simulink library "tqd"  (R2021b)
settings: Solver=VariableStepAuto  StartTime=0.0  StopTime=10.0  RelTol=1e-3
undefined symbols (not defined in the file or in its folder): ATQD_APSDecReq_X_kph, ATQD_APSDecReq_Y_mps2, ATQD_APSDecReqCMD_X_kph, ATQD_APSDecReqTs_X_pct, ATQD_APSDecTimeGain_X_Deg, ATQD_APSDecTimeGain_Y_s, ATQD_APSReqLowSpd_X_Deg, ATQD_AutoHoldReleaseBPS_X_Deg, ATQD_AWDLoadTrqnsGain_X_kg, ATQD_AWDLoadTrqnsGain_Y_pct, ATQD_BOSEnBPSPosn_X_kph, ATQD_BOSMap_X_rpm, ATQD_BOSMap_Y_pct, ATQD_CreepBaseTqD_X_kph, ATQD_CreepBaseTqD_Y_Deg, ATQD_CreepBaseTqR_X_kph, ATQD_CreepBaseTqR_Y_Deg, ATQD_CreepBPSDisPosn_X_Deg, ATQD_CreepBPSDisPosnR_X_Deg, ATQD_CreepBPSEnPosn_X_Deg, ATQD_CreepBPSEnPosnR_X_Deg, ATQD_CreepDeltaTq_X_kph, ATQD_CreepIterm_X_kph, ATQD_CreepIterm_Y_kph, ATQD_CreepItermMaxLimit_X_pct, ATQD_CreepPreloadTime_X_kph, ATQD_CreepPreloadTq_X_kph, ATQD_CreepPreloadTq_Y_s, ATQD_CreepProtTq_X_Deg, ATQD_CreepPterm_X_kph, ATQD_CreepPterm_Y_kph, ATQD_ECOTqMapD_X_rpm, ATQD_ECOTqMapD_Y_pct, ATQD_EOPDTqMapDCon_X_rpm, ATQD_EOPDTqMapDCon_Y_Deg, ATQD_EstInitVehWeight_X_c, ATQD_LHMRollGenMapD_X_rpm, ATQD_LHMRollGenMapD_Y_rpm, ATQD_LHMTqMapD_X_rpm, ATQD_LHMTqMapD_Y_pct, ATQD_NL1TqMapD_X_rpm, ATQD_NL1TqMapD_Y_pct, ATQD_NOPDTqMapDCon_X_rpm, ATQD_NOPDTqMapDCon_Y_Deg, ATQD_NRMRrEDUSpRat_X_rpm, ATQD_NRMRrEDUSpRat_Y_Nm, ATQD_OPDHoldDownRelDelay_X_Deg, ATQD_OPDHoldEnSpd_X_Deg, ATQD_OPDHoldRelDetTime_X_Deg, ATQD_OPDHoldReleaseTq_X_Deg, ATQD_OrigPedTqLowLim_X_Deg, ATQD_OrigPedTqLowLim_Y_pct, ATQD_PedalMapClimbUpLim_X_rpm, ATQD_PedalMapClimbUpLim_Y_Deg, ATQD_PreLoadTq_X_s, ATQD_RollGenMapEL1_X_rpm, ATQD_RollGenMapEL1_Y_rpm, ATQD_SL1TqMapD_X_rpm, ATQD_SL1TqMapD_Y_pct, ATQD_SlideRegenTqGain_X_Gps ... (+487)
libraries: hcu_lib x83, simulink x73, tqr x1
(part 9 of 19)

== system tqd/TQD/TorqueDemand/Signal_convert/SWC2_Subsystem/L_ScrollPress Behavior ==
  note: If press time more then Long press's limit then go Long press only. Else go short press only. Else if no press.
  note: Long press or Short press
  VTQD_SWC2LScrollPressSta_flg : Inport
  TASK_TIME : Inport  Port=2
  AND : Logic  AllPortsSameDT=off  OutDataTypeStr=boolean
  Constant10 : Constant  Value=FALSE
  Constant3 : Constant  Value=KTQD_SpdModeShortPLim_s
  Constant7 : Constant  Value=FALSE
  Default 3 sec : Constant  Value=KTQD_SpdModeLongPLim_s
  DelayEnable_LONG_PRESS : hcu_lib/Basic_Blocks/DelayEnable
  DelayEnable_SHORT_PRESS : hcu_lib/Basic_Blocks/DelayEnable
  Detect Decrease1 : simulink/Logic and Bit Operations/Detect Decrease  vinit=0.0  OutDataTypeStr=boolean
  Detect Decrease2 : simulink/Logic and Bit Operations/Detect Decrease  vinit=0.0  OutDataTypeStr=boolean
  Detect Increase : simulink/Logic and Bit Operations/Detect Increase  vinit=0.0  OutDataTypeStr=boolean
  Switch1 : Switch  Criteria=u2 > Threshold
  Switch2 : Switch  Criteria=u2 ~= 0
  VTQD_LScrollPressShort_flg : Outport
  "VTQD_LScrollPressLong_flg\t" : Outport  Port=2
  wires:
  Detect Increase/1 -> "VTQD_LScrollPressLong_flg\t"/1
  [TASK_TIME] -> DelayEnable_LONG_PRESS/3
  Default 3 sec/1 -> DelayEnable_LONG_PRESS/2
  [TASK_TIME] -> DelayEnable_SHORT_PRESS/3
  Constant3/1 -> DelayEnable_SHORT_PRESS/2
  DelayEnable_SHORT_PRESS/1 -> Detect Decrease2/1
  Constant7/1 -> Switch1/3
  DelayEnable_LONG_PRESS/1 -> Switch1/1, Switch1/2
  [Short_press_falling_Edge] -> AND/1
  [Long_press] -> Detect Decrease1/1, Detect Increase/1
  Constant10/1 -> Switch2/1
  [Short_press_falling_Edge] -> Switch2/3
  [VTQD_SWC2LScrollPressSta_flg] -> DelayEnable_SHORT_PRESS/1, DelayEnable_LONG_PRESS/1
  AND/1 -> Switch2/2
  Switch2/1 -> VTQD_LScrollPressShort_flg/1
  VTQD_SWC2LScrollPressSta_flg/1 -> [VTQD_SWC2LScrollPressSta_flg]
  Detect Decrease1/1 -> AND/2
  Detect Decrease2/1 -> [Short_press_falling_Edge]
  Switch1/1 -> [Long_press]
  TASK_TIME/1 -> [TASK_TIME]

== system tqd/TQD/TorqueDemand/Signal_convert/SWC2_Subsystem/Road Speed Limit Convert ==
  VINP_ADASSLIFSpdLim_enum : Inport
  VINP_IVIISAOffsetSpd_enum : Inport  Port=2
  VTQD_IVIISAOffsetSpdCHOOSE_flg : Inport  Port=3
  VINP_Distanceunit_flg : Inport  Port=4
  VTQD_ShiftGearPosn_enum : Inport  Port=5
  " 20" : Constant  Value=KTQD_ACCActiveMetSpdLoMPH_mph
  " 30kph" : Constant  Value=KTQD_ACCActiveMetSpdLo_kph
  AND{,1..3} (4 alike) : Logic  AllPortsSameDT=off  OutDataTypeStr=boolean
  Add{,1..3} (4 alike) : Sum  Inputs=+-
  Add4 : Sum
  Constant{,17..18,20} (4 alike) : Constant  Value=0x11  OutDataTypeStr=uint8
  Constant1 : Constant  Value=10  OutDataTypeStr=single
  Constant10 : Constant  Value=15  OutDataTypeStr=single
  Constant{11,13..15} (4 alike) : Constant  Value=ZERO_FLOAT  OutDataTypeStr=single
  Constant12 : Constant  Value=ENUM_GEARPOSNTOCAN_D  OutDataTypeStr=uint8
  Constant16 : Constant  Value=KTQD_SpdLimOffsetOn_flg  OutDataTypeStr=single
  Constant19 : Constant  Value=MPH2KPH  OutDataTypeStr=uint8
  Constant2 : Constant  Value=0x10  OutDataTypeStr=uint8
  Constant21 : Constant  Value=KPH2MPH  OutDataTypeStr=uint8
  Constant{3,7..9} (4 alike) : Constant  Value=5  OutDataTypeStr=single
  Constant4 : Constant  Value=0x0  OutDataTypeStr=uint8
  Constant5 : Constant  Value=0x9  OutDataTypeStr=uint8
  Constant6 : Constant  Value=0x9  OutDataTypeStr=uint8
  Data Type Conversion{,1..3} (4 alike) : DataTypeConversion  OutDataTypeStr=single
  Delay : Delay  DelayLength=1
  Divide : Product  Inputs=**
  Divide1 : Product  Inputs=**
  Equal : RelationalOperator  Operator=~=  OutDataTypeStr=boolean  RndMeth=Simplest
  Equal1 : RelationalOperator  Operator===  OutDataTypeStr=boolean  RndMeth=Simplest
  Max : MinMax  Function=max  Inputs=2
  NOT : Logic  Operator=NOT  AllPortsSameDT=off  OutDataTypeStr=boolean
  NOT1 : Logic  Operator=NOT  AllPortsSameDT=off  OutDataTypeStr=boolean
  Product{,1..3} (4 alike) : Product
  Relational Operator{,1,3..5} (5 alike) : RelationalOperator  OutDataTypeStr=boolean  RndMeth=Simplest
  Relational Operator2 : RelationalOperator  Operator=>  OutDataTypeStr=boolean  RndMeth=Simplest
  Switch{,1..9} (10 alike) : Switch  Criteria=u2 > Threshold
  VTQD_RoadSpdLim_raw32 : Outport
  wires:
  VINP_ADASSLIFSpdLim_enum/1 -> [VINP_ADASSLIFSpdLim_enum]
  VINP_IVIISAOffsetSpd_enum/1 -> [VINP_IVIISAOffsetSpd_enum]
  [VINP_ADASSLIFSpdLim_enum] -> Relational Operator/1
  Relational Operator/1 -> Switch/2
  Constant/1 -> Relational Operator/2
  [VINP_ADASSLIFSpdLim_enum] -> Data Type Conversion/1
  Data Type Conversion/1 -> Product/1
  Constant1/1 -> Product/2
  Product/1 -> Switch/3
  [VINP_ADASSLIFSpdLim_enum] -> Add/1
  Constant2/1 -> Add/2
  Product1/1 -> Switch/1
  Constant3/1 -> Product1/2
  Add/1 -> Data Type Conversion1/1
  Data Type Conversion1/1 -> Product1/1
  Equal/1 -> Switch1/2
  Constant4/1 -> Equal/2
  Switch/1 -> Switch1/1
  Switch5/1 -> [VTQD_CalRoadSpdLim_raw32], Delay/1  "VTQD_CalRoadSpdLim_raw32"
  [VINP_IVIISAOffsetSpd_enum] -> Relational Operator1/1
  Constant5/1 -> Relational Operator1/2
  Relational Operator1/1 -> Switch2/2
  Data Type Conversion2/1 -> Product2/1
  [VINP_IVIISAOffsetSpd_enum] -> Add1/1
  Constant6/1 -> Add1/2
  Add1/1 -> Data Type Conversion2/1
  Constant7/1 -> Product2/2
  Product2/1 -> Add2/1
  Constant8/1 -> Add2/2
  [VINP_IVIISAOffsetSpd_enum] -> Data Type Conversion3/1
  Constant9/1 -> Product3/2
  Data Type Conversion3/1 -> Product3/1
  Constant10/1 -> Add3/2
  Product3/1 -> Add3/1
  Add3/1 -> Switch2/3
  Add2/1 -> Switch2/1
  VTQD_IVIISAOffsetSpdCHOOSE_flg/1 -> [VTQD_IVIISAOffsetSpdCHOOSE_flg]
  Switch2/1 -> Switch3/1
  Constant11/1 -> Switch3/3
  Switch3/1 -> [VTQD_CalRoadSpdLimOffSet_c]  "VTQD_CalRoadSpdLimOffSet_c"
  Switch6/1 -> Add4/2
  [VTQD_CalRoadSpdLim_raw32] -> Add4/1
  [VTQD_RoadSpdLim_raw32] -> VTQD_RoadSpdLim_raw32/1
  [VTQD_IVIISAOffsetSpdCHOOSE_flg] -> AND/1
  " 20"/1 -> Switch4/1
  " 30kph"/1 -> Switch4/3
  [VINP_Distanceunit_flg] -> Switch4/2
  VINP_Distanceunit_flg/1 -> [VINP_Distanceunit_flg]
  Delay/1 -> Switch1/3
  Switch4/1 -> Max/1
  Max/1 -> [VTQD_RoadSpdLim_raw32]  "VTQD_RoadSpdLim_raw32"
  Add4/1 -> [VTQD_SpdLimAftOffset_raw32]  "VTQD_SpdLimAftOffset_raw32"
  [VINP_ADASSLIFSpdLim_enum] -> Equal/1
  Equal1/1 -> Switch5/2
  Constant12/1 -> Equal1/2
  Switch1/1 -> Switch5/1
  Constant13/1 -> Switch5/3
  VTQD_ShiftGearPosn_enum/1 -> [VTQD_ShiftGearPosn_enum]
  [VTQD_ShiftGearPosn_enum] -> Equal1/1
  [VTQD_CalRoadSpdLimOffSet_c] -> Relational Operator2/1, Switch6/1
  Relational Operator2/1 -> Switch6/2
  Constant14/1 -> Relational Operator2/2
  Constant15/1 -> Switch6/3
  AND/1 -> Switch3/2
  Constant16/1 -> AND/2
  Constant17/1 -> Relational Operator3/2
  [VINP_ADASSLIFSpdLim_enum] -> Relational Operator3/1
  Relational Operator3/1 -> AND1/2
  [VINP_Distanceunit_flg] -> AND1/1
  AND1/1 -> Switch7/2
  Switch7/1 -> Max/2
  [VTQD_SpdLimAftOffset_raw32] -> Switch7/1
  AND2/1 -> Switch8/2
  [VINP_Distanceunit_flg] -> NOT/1
  Relational Operator4/1 -> AND2/2
  [VINP_ADASSLIFSpdLim_enum] -> Relational Operator4/1
  Constant18/1 -> Relational Operator4/2
  Switch8/1 -> Switch7/3
  NOT/1 -> AND2/1
  [VTQD_SpdLimAftOffset_raw32] -> Divide/1
  Divide/1 -> Switch8/1
  Constant19/1 -> Divide/2
  AND3/1 -> Switch9/2
  [VINP_Distanceunit_flg] -> AND3/1
  Relational Operator5/1 -> NOT1/1
  [VINP_ADASSLIFSpdLim_enum] -> Relational Operator5/1
  Constant20/1 -> Relational Operator5/2
  Switch9/1 -> Switch8/3
  NOT1/1 -> AND3/2
  Constant21/1 -> Divide1/2
  [VTQD_SpdLimAftOffset_raw32] -> Divide1/1
  Divide1/1 -> Switch9/1
  [VTQD_SpdLimAftOffset_raw32] -> Switch9/3

== system tqd/TQD/TorqueDemand/Signal_convert/SWC2_Subsystem/Speed Setting Mode ==
  note: Botton logic
  note: INPUT Signal
  note: PWRSTA and DRIVE GEAR GOOD
  note: OUTPUT SET SPEED
  VPMM_PowerSta_enum : Inport
  VTQD_ShiftGearPosn_enum : Inport  Port=2
  VTQD_SpdCtrlMode_enum : Inport  Port=3
  VINP_ADASACCSta_enum : Inport  Port=4
  VVMC_CCCtrlSta_enum : Inport  Port=5
  VVMC_MSACtrlSta_enum : Inport  Port=6
  VINP_ADASSLIFSpdLim_enum : Inport  Port=7
  VTQD_SWC2ScrollUpSta_flg : Inport  Port=8
  VTQD_SWC2ScrollDownSta_flg : Inport  Port=9
  task_time_s : Inport  Port=10
  VVMC_LVDAACCStatusInformation_flg : Inport  Port=11
  VVMC_ACCObjDist_m : Inport  Port=12
  VTQD_SpdLim4SetSpd_raw32 : Inport  Port=13
  VINP_Distanceunit_flg : Inport  Port=14
  VTQD_SWC2ResUpSta_flg : Inport  Port=15
  VTQD_SWC2SetDownSta_flg : Inport  Port=16
  VINP_SmartEcoModeSW_flg : Inport  Port=17
  VVMC_SetACCDisableAPS_flg : Inport  Port=18
  VINP_IVIACCAdaptiveSta_flg : Inport  Port=19
  VTQD_Set2MeterSpd_flg : Inport  Port=20
  VTQD_SetRoadSpdLim_flg : Inport  Port=21
  VTQD_LScrollPressShort_flg : Inport  Port=22
  VVMC_MeterIndSpeed_raw32 : Inport  Port=23
  ACC Speed Setting ON : Subsystem  TreatAsAtomicUnit=on
  AND{,1..3,5,8} (6 alike) : Logic  AllPortsSameDT=off  OutDataTypeStr=boolean
  AND6 : Logic  Inputs=3  AllPortsSameDT=off  OutDataTypeStr=boolean
  AND7 : Logic  Operator=OR  AllPortsSameDT=off  OutDataTypeStr=boolean
  CC Speed Setting ON : Subsystem  TreatAsAtomicUnit=on
  Constant : Constant  Value=ZERO_INT
  Constant1 : Constant  Value=ENUM_SPDCTRLMODE_CC
  Constant10 : Constant  Value=ENUM_SPDCTRLMODE_ISA
  Constant11 : Constant  Value=ENUM_SPDCTRLMODE_OFF
  Constant12 : Constant  Value=KTQD_SetSpdDeltaLongFit_kph
  Constant13 : Constant  Value=ZERO_INT
  Constant14 : Constant  Value=KTQD_SmartEcoLimitSpd_kph
  Constant15 : Constant  Value=KTQD_SmartEcoLimitSpd_mph
  Constant16 : Constant  Value=KTQD_SmartEcoLimitSpd_kph
  Constant17 : Constant  Value=KTQD_SmartEcoLimitSpd_mph
  Constant18 : Constant  Value=KTQD_SmartEcoLimitSpd_kph
  Constant19 : Constant  Value=KTQD_SmartEcoLimitSpd_mph
  Constant2 : Constant  Value=ENUM_POWERSTA_READY
  Constant3 : Constant  Value=ENUM_SPDCTRLMODE_ACC
  Constant4 : Constant  Value=ENUM_GEARPOSNTOCAN_D
  Constant5 : Constant  Value=ENUM_SPDCTRLMODE_MSA
  Constant6 : Constant  Value=ENUM_SPDCTRLMODE_ISA
  Constant7 : Constant  Value=ENUM_SPDCTRLMODE_ACC
  Constant8 : Constant  Value=ENUM_SPDCTRLMODE_CC
  Constant9 : Constant  Value=ENUM_SPDCTRLMODE_MSA
  Data Type Conversion : DataTypeConversion  OutDataTypeStr=uint8
  Delay : Delay  DelayLength=1
  Else Speed Setting On : Subsystem  TreatAsAtomicUnit=on
  Equal{1..11} (11 alike) : RelationalOperator  Operator===  OutDataTypeStr=boolean  RndMeth=Simplest
  ISA Speed Setting ON : Subsystem  TreatAsAtomicUnit=on
  If : If  NumInputs=4  IfExpression=u1 ~= 0  ElseIfExpressions=u2 ~= 0, u3~= 0, u4~= 0
  MSA Speed Setting ON : Subsystem  TreatAsAtomicUnit=on
  OR : Logic  Operator=OR  AllPortsSameDT=off  OutDataTypeStr=boolean
  Relational Operator : RelationalOperator  OutDataTypeStr=boolean  RndMeth=Simplest
  Relational Operator1 : RelationalOperator  OutDataTypeStr=boolean  RndMeth=Simplest
  Relational Operator2 : RelationalOperator  OutDataTypeStr=boolean  RndMeth=Simplest
  Rem : Math  Operator=rem  SaturateOnIntegerOverflow=on
  SWC2ScrollDownSta : Subsystem
  SWC2ScrollUpSta : Subsystem
  Switch{,1..4} (5 alike) : Switch  Criteria=u2 ~= 0
  Switch5 : Switch  Criteria=u2 > Threshold
  Switch6 : Switch  Criteria=u2 > Threshold
  Switch7 : Switch  Criteria=u2 > Threshold
  VTQD_SetSpd_kph : Outport
  VTQD_SWC2ScrollUpSta_enum : Outport  Port=2
  VTQD_SWC2SetSpdLimWarn_flg : Outport  Port=3
  VTQD_SWC2ACCSetSpd_kph : Outport  Port=4
  VTQD_SWC2CCSetSpd_kph : Outport  Port=5
  VTQD_SWC2MSASetSpd_kph : Outport  Port=6
  VTQD_SWC2ISASetSpd_kph : Outport  Port=7
  VTQD_SWC2AllowSetSpd_flg : Outport  Port=8
  VTQD_SWC2CCSpdResetFinish_flg : Outport  Port=9
  wires:
  MSA Speed Setting ON/1(VSCP_MSASetSpd_kph) -> VTQD_SWC2MSASetSpd_kph/1, [VTQD_MSASetSpd_kph]  "VTQD_SWC2MSASetSpd_kph"
  CC Speed Setting ON/1(VTQD_CCSetSpd_kph) -> [VTQD_CCSetSpd_kph], VTQD_SWC2CCSetSpd_kph/1  "VTQD_SWC2CCSetSpd_kph"
  VVMC_CCCtrlSta_enum/1 -> [VVMC_CCCtrlSta_enum]
  VINP_ADASSLIFSpdLim_enum/1 -> [VINP_ADASSLIFSpdLim_enum]
  task_time_s/1 -> [task_time_s]
  Switch/1 -> [VTQD_SetSpd_kph], VTQD_SetSpd_kph/1  "VTQD_SetSpd_kph"
  Constant/1 -> Switch4/1
  Switch4/1 -> Switch3/3
  Equal11/1 -> Switch4/2
  [VTQD_SpdCtrlMode_enum] -> Equal11/1
  Constant11/1 -> Equal11/2
  Switch3/1 -> Switch2/3
  Constant10/1 -> Equal10/2
  [VTQD_SpdCtrlMode_enum] -> Equal10/1
  Equal10/1 -> Switch3/2
  [VTQD_ISASetSpd_kph] -> Switch3/1
  Switch2/1 -> Switch1/3
  [VTQD_MSASetSpd_kph] -> Switch2/1
  Equal9/1 -> Switch2/2
  [VTQD_SpdCtrlMode_enum] -> Equal9/1
  Constant9/1 -> Equal9/2
  Switch1/1 -> Switch/3
  Constant8/1 -> Equal8/2
  [VTQD_SpdCtrlMode_enum] -> Equal8/1
  Equal8/1 -> Switch1/2
  [VTQD_CCSetSpd_kph] -> Switch1/1
  [VTQD_ACCSetSpd_kph] -> Switch/1
  Equal7/1 -> Switch/2
  [VTQD_SpdCtrlMode_enum] -> Equal7/1
  Constant7/1 -> Equal7/2
  ISA Speed Setting ON/1(VTQD_ISASetSpd_kph) -> VTQD_SWC2ISASetSpd_kph/1, [VTQD_ISASetSpd_kph]  "VTQD_SWC2ISASetSpd_kph"
  If/5 -> Else Speed Setting On/Action
  If/4 -> ISA Speed Setting ON/Action
  AND5/1 -> If/4
  [VTQD_PwrstaANDGearRdy_flg] -> AND5/1
  [VTQD_SpdCtrlMode_enum] -> Equal6/1
  Constant6/1 -> Equal6/2
  Equal6/1 -> AND5/2
  VVMC_MSACtrlSta_enum/1 -> [VVMC_MSACtrlSta_enum]
  Equal5/1 -> If/3
  Constant5/1 -> Equal5/2
  [VTQD_SpdCtrlMode_enum] -> Equal5/1
  If/3 -> MSA Speed Setting ON/Action
  [VVMC_MSACtrlSta_enum] -> MSA Speed Setting ON/1(VVMC_MSACrlSta_enum)
  If/2 -> CC Speed Setting ON/Action
  [VTQD_SWC2ScrollDownSta_enum] -> CC Speed Setting ON/3("VTQD_SWCSetDownPress_enum  ")
  [VTQD_SWC2ScrollUpSta_enum] -> CC Speed Setting ON/2("VTQD_SWCResUpPress_enum  ")
  [VVMC_CCCtrlSta_enum] -> CC Speed Setting ON/1(VVMC_CCCtrlSta_enum)
  VINP_ADASACCSta_enum/1 -> [VINP_ADASACCSta_enum]
  VTQD_SWC2ScrollDownSta_flg/1 -> [VTQD_SWC2ScrollDownSta_flg]
  VTQD_SWC2ScrollUpSta_flg/1 -> [VTQD_SWC2ScrollUpSta_flg]
  AND3/1 -> If/2
  [VTQD_PwrstaANDGearRdy_flg] -> AND3/1
  [VTQD_SpdCtrlMode_enum] -> Equal1/1
  Constant1/1 -> Equal1/2
  Equal1/1 -> AND3/2
  AND2/1 -> [VTQD_PwrstaANDGearRdy_flg]
  [VPMM_PowerSta_enum] -> Equal2/1
  Constant2/1 -> Equal2/2
  [VTQD_ShiftGearPosn_enum] -> Equal4/1
  Constant4/1 -> Equal4/2
  Equal2/1 -> AND2/1
  Equal4/1 -> AND2/2
  AND1/1 -> If/1
  Equal3/1 -> AND1/2
  Constant3/1 -> Equal3/2
  [VTQD_SpdCtrlMode_enum] -> Equal3/1
  If/1 -> ACC Speed Setting ON/Action
  VTQD_SpdCtrlMode_enum/1 -> [VTQD_SpdCtrlMode_enum]
  [VTQD_PwrstaANDGearRdy_flg] -> AND1/1
  VTQD_ShiftGearPosn_enum/1 -> [VTQD_ShiftGearPosn_enum]
  VPMM_PowerSta_enum/1 -> [VPMM_PowerSta_enum]
  [VINP_ADASSLIFSpdLim_enum] -> ISA Speed Setting ON/1(VINP_ADASSLIFSpdLim_enum)
  [VTQD_SWC2ScrollUpSta_flg] -> SWC2ScrollUpSta/1(INPUT)
  SWC2ScrollUpSta/1(OUTPUT) -> VTQD_SWC2ScrollUpSta_enum/1, [VTQD_SWC2ScrollUpSta_enum]  "VTQD_SWC2ScrollUpSta_enum"
  [task_time_s] -> SWC2ScrollDownSta/2(task_time_s)
  [VTQD_SWC2ScrollDownSta_flg] -> SWC2ScrollDownSta/1(INPUT)
  SWC2ScrollDownSta/1(OUTPUT) -> [VTQD_SWC2ScrollDownSta_enum]  "VTQD_SWC2ScrollDownSta_enum"
  [task_time_s] -> SWC2ScrollUpSta/2(task_time_s)
  Rem/1 -> Data Type Conversion/1
  Data Type Conversion/1 -> [VTQD_SetSpdDeltaLongFit_kph]
  [VTQD_SetSpd_kph] -> Delay/1
  Delay/1 -> Rem/1
  Constant12/1 -> Rem/2
  [VTQD_SetSpdDeltaLongFit_kph] -> CC Speed Setting ON/5(VTQD_SetSpdDeltaLongFit_kph)
  [VTQD_SpdLim4SetSpd_raw32] -> CC Speed Setting ON/4(VTQD_SpdLim4SetSpd_raw32)
  [VTQD_SpdLim4SetSpd_raw32] -> MSA Speed Setting ON/4(VTQD_SpdLim4SetSpd_raw32)
  [VTQD_SetSpdDeltaLongFit_kph] -> MSA Speed Setting ON/5(VTQD_SetSpdDeltaLongFit_kph)
  Constant13/1 -> Else Speed Setting On/1(In)
  Else Speed Setting On/1(Out) -> [VTQD_ElseSetSpd_kph]
  [VTQD_ElseSetSpd_kph] -> Switch4/3
  [VINP_ADASACCSta_enum] -> ACC Speed Setting ON/7(VINP_ADASACCSta_enum)
  [VTQD_SpdLim4SetSpd_raw32] -> ACC Speed Setting ON/6(VTQD_SpdLim4SetSpd_raw32)
  [task_time_s] -> ACC Speed Setting ON/3(task_time_s)
  ACC Speed Setting ON/1(VTQD_ACCSetSpd_kph) -> [VTQD_ACCSetSpd_kph], VTQD_SWC2ACCSetSpd_kph/1  "VTQD_SWC2ACCSetSpd_kph"
  VTQD_SpdLim4SetSpd_raw32/1 -> [VTQD_SpdLim4SetSpd_raw32]
  VINP_Distanceunit_flg/1 -> [VINP_Distanceunit_flg]
  [VINP_Distanceunit_flg] -> ACC Speed Setting ON/8(VINP_Distanceunit_flg)
  [VINP_Distanceunit_flg] -> CC Speed Setting ON/6(VINP_Distanceunit_flg)
  [VINP_Distanceunit_flg] -> MSA Speed Setting ON/6(VINP_Distanceunit_flg)
  VTQD_SWC2ResUpSta_flg/1 -> [VTQD_SWC2ResUpSta_flg]
  VTQD_SWC2SetDownSta_flg/1 -> [VTQD_SWC2SetDownSta_flg]
  [VTQD_SWC2ResUpSta_flg] -> ACC Speed Setting ON/9(VTQD_SWC2ResUpSta_flg)
  [VTQD_SWC2SetDownSta_flg] -> ACC Speed Setting ON/10(VTQD_SWC2SetDownSta_flg)
  [VTQD_SWC2ScrollDownSta_enum] -> ACC Speed Setting ON/2(VTQD_SWC2ScrollDownSta_enum)
  [VTQD_SWC2ScrollUpSta_enum] -> ACC Speed Setting ON/1(VTQD_SWC2ScrollUpSta_enum)
  [VTQD_SWC2ScrollUpSta_enum] -> MSA Speed Setting ON/2("VTQD_SWC2ScrollUpSta_enum  ")
  [VTQD_SWC2ScrollDownSta_enum] -> MSA Speed Setting ON/3("VTQD_SWC2ScrollDownSta_enum  ")
  [VTQD_SWC2ResUpSta_flg] -> MSA Speed Setting ON/7(VTQD_SWC2ResUpSta_flg)
  [VTQD_SWC2SetDownSta_flg] -> MSA Speed Setting ON/8(VTQD_SWC2SetDownSta_flg)
  VINP_SmartEcoModeSW_flg/1 -> [VINP_SmartEcoModeSW_flg]
  [VINP_SmartEcoModeSW_flg] -> ACC Speed Setting ON/11(VINP_SmartEcoModeSW_flg)
  [VINP_SmartEcoModeSW_flg] -> CC Speed Setting ON/7(VINP_SmartEcoModeSW_flg)
  [VINP_SmartEcoModeSW_flg] -> MSA Speed Setting ON/9(VINP_SmartEcoModeSW_flg)
  [VINP_SmartEcoModeSW_flg] -> ISA Speed Setting ON/2(VINP_SmartEcoModeSW_flg)
  AND7/1 -> AND8/1
  OR/1 -> AND6/2
  Relational Operator1/1 -> AND6/1
  [VINP_SmartEcoModeSW_flg] -> AND8/2
  Relational Operator/1 -> AND/1
  Relational Operator2/1 -> AND6/3
  Switch6/1 -> Relational Operator1/2
  Switch7/1 -> Relational Operator2/2
  AND8/1 -> VTQD_SWC2SetSpdLimWarn_flg/1
  AND6/1 -> AND7/2
  AND/1 -> AND7/1
  Switch5/1 -> Relational Operator/2
  [VTQD_SetSpd_kph] -> Relational Operator/1
  Constant15/1 -> Switch5/1
  [VINP_Distanceunit_flg] -> Switch5/2
  Constant14/1 -> Switch5/3
  Constant17/1 -> Switch6/1
  [VINP_Distanceunit_flg] -> Switch6/2
  Constant16/1 -> Switch6/3
  [VTQD_SetSpd_kph] -> Relational Operator2/1
  Constant19/1 -> Switch7/1
  [VINP_Distanceunit_flg] -> Switch7/2
  Constant18/1 -> Switch7/3
  [VTQD_SpdLim4SetSpd_raw32] -> Relational Operator1/1
  [VTQD_SWC2ResUpSta_flg] -> OR/1
  [VTQD_SWC2SetDownSta_flg] -> OR/2
  [VTQD_SWC2ScrollUpSta_flg] -> AND/2
  VINP_IVIACCAdaptiveSta_flg/1 -> [VINP_IVIACCAdaptiveSta_flg]
  [VTQD_Set2MeterSpd_flg] -> ACC Speed Setting ON/14(VTQD_Set2MeterSpd_flg)
  [VTQD_SetRoadSpdLim_flg] -> ACC Speed Setting ON/15(VTQD_SetRoadSpdLim_flg)
  [VINP_ADASSLIFSpdLim_enum] -> ACC Speed Setting ON/16(VINP_ADASSLIFSpdLim_enum)
  [VTQD_LScrollPressShort_flg] -> ACC Speed Setting ON/17(VTQD_LScrollPressShort_flg)
  [VINP_IVIACCAdaptiveSta_flg] -> ACC Speed Setting ON/13(VINP_IVIACCAdaptiveSta_flg)
  VTQD_Set2MeterSpd_flg/1 -> [VTQD_Set2MeterSpd_flg]
  VTQD_SetRoadSpdLim_flg/1 -> [VTQD_SetRoadSpdLim_flg]
  VTQD_LScrollPressShort_flg/1 -> [VTQD_LScrollPressShort_flg]
  [VINP_IVIACCAdaptiveSta_flg] -> MSA Speed Setting ON/10(VINP_IVIACCAdaptiveSta_flg)
  [VTQD_Set2MeterSpd_flg] -> MSA Speed Setting ON/11(VTQD_Set2MeterSpd_flg)
  [VTQD_SetRoadSpdLim_flg] -> MSA Speed Setting ON/12(VTQD_SetRoadSpdLim_flg)
  [VINP_ADASSLIFSpdLim_enum] -> MSA Speed Setting ON/13(VINP_ADASSLIFSpdLim_enum)
  [VTQD_LScrollPressShort_flg] -> MSA Speed Setting ON/14(VTQD_LScrollPressShort_flg)
  VVMC_MeterIndSpeed_raw32/1 -> [VVMC_MeterIndSpeed_raw32]
  [VVMC_MeterIndSpeed_raw32] -> ACC Speed Setting ON/18(VVMC_MeterIndSpeed_raw32)
  [VVMC_MeterIndSpeed_raw32] -> MSA Speed Setting ON/15(VVMC_MeterIndSpeed_raw32)
  VVMC_SetACCDisableAPS_flg/1 -> [VVMC_SetACCDisableAPS_flg]
  [VVMC_SetACCDisableAPS_flg] -> ACC Speed Setting ON/12(VVMC_SetACCDisableAPS_flg)
  VVMC_LVDAACCStatusInformation_flg/1 -> [VVMC_LVDAACCStatusInformation_flg]
  VVMC_ACCObjDist_m/1 -> [VVMC_ACCObjDist_m]
  [VVMC_ACCObjDist_m] -> ACC Speed Setting ON/5(VVMC_ACCObjDist_m)
  [VVMC_LVDAACCStatusInformation_flg] -> ACC Speed Setting ON/4(VVMC_LVDAACCStatusInformation_flg)
  ACC Speed Setting ON/2(VTQD_SWC2AllowSetSpd_flg) -> VTQD_SWC2AllowSetSpd_flg/1
  CC Speed Setting ON/2(VTQD_SWC2CCSpdResetFinish_flg) -> VTQD_SWC2CCSpdResetFinish_flg/1

== system tqd/TQD/TorqueDemand/Signal_convert/SWC2_Subsystem/VTQD_IVIISAOffsetSpdCHOOSE_flg ==
  VTQD_IVIISAOffsetSpd_enum : Inport
  Constant : Constant  Value=ENUM_IVIISAOFFSETSPD_MIUNS10KPH
  Constant1 : Constant  Value=ENUM_IVIISAOFFSETSPD_MIUNS5KPH
  Constant2 : Constant  Value=ENUM_IVIISAOFFSETSPD_0KPH
  Constant3 : Constant  Value=ENUM_IVIISAOFFSETSPD_PLUS5KPH
  Constant4 : Constant  Value=ENUM_IVIISAOFFSETSPD_PLUS10KPH
  Constant5 : Constant  Value=ENUM_IVIISAOFFSETSPD_MIUNS5MPH
  Constant6 : Constant  Value=ENUM_IVIISAOFFSETSPD_0MPH
  Constant7 : Constant  Value=ENUM_IVIISAOFFSETSPD_PLUS5MPH
  Constant8 : Constant  Value=TRUE
  Constant9 : Constant  Value=FALSE
  Equal{,1..7} (8 alike) : RelationalOperator  Operator===  OutDataTypeStr=boolean  RndMeth=Simplest
  OR : Logic  Operator=OR  Inputs=8  AllPortsSameDT=off  OutDataTypeStr=boolean
  Switch : Switch  Criteria=u2 ~= 0
  VTQD_IVIISAOffsetSpdCHOOSE_flg : Outport
  wires:
  VTQD_IVIISAOffsetSpd_enum/1 -> [VTQD_IVIISAOffsetSpd_enum], Equal/1
  Constant/1 -> Equal/2
  Equal/1 -> OR/1
  Constant1/1 -> Equal1/2
  Equal1/1 -> OR/2
  Equal2/1 -> OR/3
  Constant2/1 -> Equal2/2
  Constant5/1 -> Equal5/2
  Equal5/1 -> OR/6
  Equal4/1 -> OR/5
  Constant4/1 -> Equal4/2
  Equal3/1 -> OR/4
  Constant3/1 -> Equal3/2
  Equal6/1 -> OR/7
  Constant6/1 -> Equal6/2
  Constant7/1 -> Equal7/2
  Equal7/1 -> OR/8
  OR/1 -> Switch/2
  Constant8/1 -> Switch/1
  Constant9/1 -> Switch/3
  Switch/1 -> VTQD_IVIISAOffsetSpdCHOOSE_flg/1  "VTQD_IVIISAOffsetSpdCHOOSE_flg"
  [VTQD_IVIISAOffsetSpd_enum] -> Equal1/1
  [VTQD_IVIISAOffsetSpd_enum] -> Equal2/1
  [VTQD_IVIISAOffsetSpd_enum] -> Equal4/1
  [VTQD_IVIISAOffsetSpd_enum] -> Equal6/1
  [VTQD_IVIISAOffsetSpd_enum] -> Equal5/1
  [VTQD_IVIISAOffsetSpd_enum] -> Equal7/1
  [VTQD_IVIISAOffsetSpd_enum] -> Equal3/1

== system tqd/TQD/TorqueDemand/Signal_convert/SWC2_Subsystem/Vehicle to Meter Speed ==
  InputSpeed : Inport
  Add : Sum
  Constant1 : Constant  Value=KTQD_Veh2MetSpdAdd_kph
  Constant11 : Constant  Value=KTQD_Veh2MetSpdGain_c
  Product : Product
  OutputSpeed : Outport
  wires:
  Constant1/1 -> Add/2
  Add/1 -> OutputSpeed/1
  Constant11/1 -> Product/2
  Product/1 -> Add/1
  InputSpeed/1 -> Product/1

== system tqd/TQD/TorqueDemand/Signal_convert/SWC_Subsystem/SpdCtrlBotton Behavior ==
  note: If press time more then Long press's limit then go Long press only. Else go short press only. Else if no press.
  note: Long press or Short press
  SWC_ACC_Sta : Inport
  TASK_TIME : Inport  Port=2
  AND : Logic  AllPortsSameDT=off  OutDataTypeStr=boolean
  Constant10 : Constant  Value=FALSE
  Constant3 : Constant  Value=KTQD_SpdModeShortPLim_s
  Constant7 : Constant  Value=FALSE
  Default 3 sec : Constant  Value=KTQD_SpdModeLongPLim_s
  DelayEnable_LONG_PRESS : hcu_lib/Basic_Blocks/DelayEnable
  DelayEnable_SHORT_PRESS : hcu_lib/Basic_Blocks/DelayEnable
  Detect Decrease1 : simulink/Logic and Bit Operations/Detect Decrease  vinit=0.0  OutDataTypeStr=boolean
  Detect Decrease2 : simulink/Logic and Bit Operations/Detect Decrease  vinit=0.0  OutDataTypeStr=boolean
  Detect Increase : simulink/Logic and Bit Operations/Detect Increase  vinit=0.0  OutDataTypeStr=boolean
  Switch1 : Switch  Criteria=u2 > Threshold
  Switch2 : Switch  Criteria=u2 ~= 0
  VTQD_SpdCtrlShortP_flg : Outport
  "VTQD_SpdCtrlLongP_flg\t" : Outport  Port=2
  wires:
  Detect Increase/1 -> "VTQD_SpdCtrlLongP_flg\t"/1
  [TASK_TIME] -> DelayEnable_LONG_PRESS/3
  Default 3 sec/1 -> DelayEnable_LONG_PRESS/2
  [TASK_TIME] -> DelayEnable_SHORT_PRESS/3
  Constant3/1 -> DelayEnable_SHORT_PRESS/2
  DelayEnable_SHORT_PRESS/1 -> Detect Decrease2/1
  Constant7/1 -> Switch1/3
  DelayEnable_LONG_PRESS/1 -> Switch1/1, Switch1/2
  [Short_press_falling_Edge] -> AND/1
  [Long_press] -> Detect Decrease1/1, Detect Increase/1
  Constant10/1 -> Switch2/1
  [Short_press_falling_Edge] -> Switch2/3
  [SWC_ACC_Sta] -> DelayEnable_SHORT_PRESS/1, DelayEnable_LONG_PRESS/1
  AND/1 -> Switch2/2
  Switch2/1 -> VTQD_SpdCtrlShortP_flg/1
  SWC_ACC_Sta/1 -> [SWC_ACC_Sta]
  Detect Decrease1/1 -> AND/2
  Detect Decrease2/1 -> [Short_press_falling_Edge]
  Switch1/1 -> [Long_press]
  TASK_TIME/1 -> [TASK_TIME]

== system tqd/TQD/TorqueDemand/Signal_convert/SWC_Subsystem/Speed Setting Mode ==
  note: Botton logic
  note: INPUT Signal
  note: PWRSTA and DRIVE GEAR GOOD
  note: OUTPUT SET SPEED
  VPMM_PowerSta_enum : Inport
  VTQD_ShiftGearPosn_enum : Inport  Port=2
  VINP_VehSpeed_kph : Inport  Port=3
  VTQD_SpdCtrlMode_enum : Inport  Port=4
  VINP_ADASACCSta_enum : Inport  Port=5
  VVMC_CCCtrlSta_enum : Inport  Port=6
  VVMC_MSACtrlSta_enum : Inport  Port=7
  VINP_ADASVehSpdLim_kph : Inport  Port=8
  VTQD_SWCResUpSta_flg : Inport  Port=9
  VTQD_SWCSetDownSta_flg : Inport  Port=10
  VTQD_SWCCancelSta_flg : Inport  Port=11
  task_time_s : Inport  Port=12
  VVMC_LVDAACCStatusInformation_flg : Inport  Port=13
  VVMC_ACCObjDist_m : Inport  Port=14
  VVMC_MeterIndSpeed_raw32 : Inport  Port=15
  VINP_Distanceunit_flg : Inport  Port=16
  VINP_SmartEcoModeSW_flg : Inport  Port=17
  VVMC_SetACCDisableAPS_flg : Inport  Port=18
  ACC Speed Setting ON : Subsystem  TreatAsAtomicUnit=on
  AND{,1..5,8} (7 alike) : Logic  AllPortsSameDT=off  OutDataTypeStr=boolean
  AND6 : Logic  Inputs=3  AllPortsSameDT=off  OutDataTypeStr=boolean
  AND7 : Logic  Operator=OR  AllPortsSameDT=off  OutDataTypeStr=boolean
  CC Speed Setting ON : Subsystem  TreatAsAtomicUnit=on
  Constant : Constant  Value=ZERO_INT
  Constant1 : Constant  Value=ENUM_SPDCTRLMODE_CC
  Constant10 : Constant  Value=ENUM_SPDCTRLMODE_ISA
  Constant11 : Constant  Value=ENUM_SPDCTRLMODE_OFF
  Constant12 : Constant  Value=KTQD_SetSpdDeltaLongFit_kph
  Constant13 : Constant  Value=ZERO_INT
  Constant14 : Constant  Value=KTQD_SmartEcoLimitSpd_kph
  Constant15 : Constant  Value=KTQD_SmartEcoLimitSpd_mph
  Constant16 : Constant  Value=KTQD_SmartEcoLimitSpd_kph
  Constant17 : Constant  Value=KTQD_SmartEcoLimitSpd_mph
  Constant18 : Constant  Value=KTQD_SmartEcoLimitSpd_kph
  Constant19 : Constant  Value=KTQD_SmartEcoLimitSpd_mph
  Constant2 : Constant  Value=ENUM_POWERSTA_READY
  Constant3 : Constant  Value=ENUM_SPDCTRLMODE_ACC
  Constant4 : Constant  Value=ENUM_GEARPOSNTOCAN_D
  Constant5 : Constant  Value=ENUM_SPDCTRLMODE_MSA
  Constant6 : Constant  Value=ENUM_SPDCTRLMODE_ISA
  Constant7 : Constant  Value=ENUM_SPDCTRLMODE_ACC
  Constant8 : Constant  Value=ENUM_SPDCTRLMODE_CC
  Constant9 : Constant  Value=ENUM_SPDCTRLMODE_MSA
  Data Type Conversion : DataTypeConversion  OutDataTypeStr=uint8
  Delay : Delay  DelayLength=1
  Else Speed Setting On : Subsystem  TreatAsAtomicUnit=on
  Equal{1..11} (11 alike) : RelationalOperator  Operator===  OutDataTypeStr=boolean  RndMeth=Simplest
  ISA Speed Setting ON : Subsystem  TreatAsAtomicUnit=on
  If : If  NumInputs=4  IfExpression=u1 ~= 0  ElseIfExpressions=u2 ~= 0, u3~= 0, u4~= 0
  MSA Speed Setting ON : Subsystem  TreatAsAtomicUnit=on
  OR : Logic  Operator=OR  AllPortsSameDT=off  OutDataTypeStr=boolean
  Relational Operator : RelationalOperator  OutDataTypeStr=boolean  RndMeth=Simplest
  Relational Operator1 : RelationalOperator  OutDataTypeStr=boolean  RndMeth=Simplest
  Relational Operator2 : RelationalOperator  OutDataTypeStr=boolean  RndMeth=Simplest
  Rem : Math  Operator=rem  SaturateOnIntegerOverflow=on
  Switch{,1..4} (5 alike) : Switch  Criteria=u2 ~= 0
  Switch5 : Switch  Criteria=u2 > Threshold
  Switch6 : Switch  Criteria=u2 > Threshold
  Switch7 : Switch  Criteria=u2 > Threshold
  VTQD_SWCCancelP_flg : Subsystem
  VTQD_SWCResUpPress_enum : Subsystem
  VTQD_SWCSetDownPress_enum : Subsystem
  VTQD_SetSpd_kph : Outport
  VTQD_SetSpdLimWarn_flg : Outport  Port=2
  VTQD_SWCACCSetSpd_kph : Outport  Port=3
  VTQD_SWCCCSetSpd_kph : Outport  Port=4
  VTQD_SWCMSASetSpd_kph : Outport  Port=5
  VTQD_SWCISASetSpd_kph : Outport  Port=6
  VTQD_SWCAllowSetSpd_flg : Outport  Port=7
  VTQD_SWCCCSpdResetFinish_flg : Outport  Port=8
  wires:
  MSA Speed Setting ON/1(VSCP_MSASetSpd_kph) -> VTQD_SWCMSASetSpd_kph/1, [VTQD_MSASetSpd_kph]  "VTQD_SWCMSASetSpd_kph"
  CC Speed Setting ON/1(VTQD_CCSetSpd_kph) -> VTQD_SWCCCSetSpd_kph/1, [VTQD_CCSetSpd_kph]  "VTQD_SWCCCSetSpd_kph"
  VVMC_CCCtrlSta_enum/1 -> [VVMC_CCCtrlSta_enum]
  VINP_ADASVehSpdLim_kph/1 -> [VINP_ADASVehSpdLim_kph]
  task_time_s/1 -> [task_time_s]
  Switch/1 -> [VTQD_SetSpd_kph], VTQD_SetSpd_kph/1
  Constant/1 -> Switch4/1
  Switch4/1 -> Switch3/3
  Equal11/1 -> Switch4/2
  [VTQD_SpdCtrlMode_enum] -> Equal11/1
  Constant11/1 -> Equal11/2
  Switch3/1 -> Switch2/3
  Constant10/1 -> Equal10/2
  [VTQD_SpdCtrlMode_enum] -> Equal10/1
  Equal10/1 -> Switch3/2
  [VTQD_ISASetSpd_kph] -> Switch3/1
  Switch2/1 -> Switch1/3
  [VTQD_MSASetSpd_kph] -> Switch2/1
  Equal9/1 -> Switch2/2
  [VTQD_SpdCtrlMode_enum] -> Equal9/1
  Constant9/1 -> Equal9/2
  Switch1/1 -> Switch/3
  Constant8/1 -> Equal8/2
  [VTQD_SpdCtrlMode_enum] -> Equal8/1
  Equal8/1 -> Switch1/2
  [VTQD_CCSetSpd_kph] -> Switch1/1
  [VTQD_ACCSetSpd_kph] -> Switch/1
  Equal7/1 -> Switch/2
  [VTQD_SpdCtrlMode_enum] -> Equal7/1
  Constant7/1 -> Equal7/2
  ISA Speed Setting ON/1(VTQD_ISASetSpd_kph) -> VTQD_SWCISASetSpd_kph/1, [VTQD_ISASetSpd_kph]  "VTQD_SWCISASetSpd_kph"
  If/5 -> Else Speed Setting On/Action
  If/4 -> ISA Speed Setting ON/Action
  AND5/1 -> If/4
  [VTQD_PwrstaANDGearGOOD_flg] -> AND5/1
  [VTQD_SpdCtrlMode_enum] -> Equal6/1
  Constant6/1 -> Equal6/2
  Equal6/1 -> AND5/2
  VVMC_MSACtrlSta_enum/1 -> [VVMC_MSACtrlSta_enum]
  AND4/1 -> If/3
  Equal5/1 -> AND4/2
  Constant5/1 -> Equal5/2
  [VTQD_SpdCtrlMode_enum] -> Equal5/1
  [VTQD_PwrstaANDGearGOOD_flg] -> AND4/1
  If/3 -> MSA Speed Setting ON/Action
  [VVMC_MSACtrlSta_enum] -> MSA Speed Setting ON/1(VVMC_MSACrlSta_enum)
  If/2 -> CC Speed Setting ON/Action
  [VTQD_SWCSetDownPress_enum] -> CC Speed Setting ON/3("VTQD_SWCSetDownPress_enum  ")
  [VTQD_SWCResUpPress_enum] -> CC Speed Setting ON/2("VTQD_SWCResUpPress_enum  ")
  [VVMC_CCCtrlSta_enum] -> CC Speed Setting ON/1(VVMC_CCCtrlSta_enum)
  VTQD_SWCCancelSta_flg/1 -> [VTQD_SWCCancelSta_flg]
  VINP_ADASACCSta_enum/1 -> [VINP_ADASACCSta_enum]
  VINP_VehSpeed_kph/1 -> [VINP_VehSpeed_kph]
  VTQD_SWCSetDownSta_flg/1 -> [VTQD_SWCSetDownSta_flg]
  VTQD_SWCResUpSta_flg/1 -> [VTQD_SWCResUpSta_flg]
  AND3/1 -> If/2
  [VTQD_PwrstaANDGearGOOD_flg] -> AND3/1
  [VTQD_SpdCtrlMode_enum] -> Equal1/1
  Constant1/1 -> Equal1/2
  Equal1/1 -> AND3/2
  AND2/1 -> [VTQD_PwrstaANDGearGOOD_flg]
  [VPMM_PowerSta_enum] -> Equal2/1
  Constant2/1 -> Equal2/2
  [VTQD_ShiftGearPosn_enum] -> Equal4/1
  Constant4/1 -> Equal4/2
  Equal2/1 -> AND2/1
  Equal4/1 -> AND2/2
  AND1/1 -> If/1
  Equal3/1 -> AND1/2
  Constant3/1 -> Equal3/2
  [VTQD_SpdCtrlMode_enum] -> Equal3/1
  If/1 -> ACC Speed Setting ON/Action
  VTQD_SpdCtrlMode_enum/1 -> [VTQD_SpdCtrlMode_enum]
  [VTQD_PwrstaANDGearGOOD_flg] -> AND1/1
  VTQD_ShiftGearPosn_enum/1 -> [VTQD_ShiftGearPosn_enum]
  VPMM_PowerSta_enum/1 -> [VPMM_PowerSta_enum]
  [VINP_ADASVehSpdLim_kph] -> ISA Speed Setting ON/1(VINP_ADASVehSpdLim_kph)
  [VTQD_SWCResUpSta_flg] -> VTQD_SWCResUpPress_enum/1(INPUT)
  VTQD_SWCResUpPress_enum/1(OUTPUT) -> [VTQD_SWCResUpPress_enum]  "VTQD_SWCResUpPress_enum"
  [task_time_s] -> VTQD_SWCSetDownPress_enum/2(task_time_s)
  [VTQD_SWCSetDownSta_flg] -> VTQD_SWCSetDownPress_enum/1(INPUT)
  VTQD_SWCSetDownPress_enum/1(OUTPUT) -> [VTQD_SWCSetDownPress_enum]  "VTQD_SWCSetDownPress_enum"
  [task_time_s] -> VTQD_SWCResUpPress_enum/2(task_time_s)
  VTQD_SWCCancelP_flg/1(Falling_edge) -> [VTQD_SWCCancelP_flg]  "VTQD_SWCCancelP_flg"
  [VTQD_SWCCancelSta_flg] -> VTQD_SWCCancelP_flg/1(INPUT)
  [VTQD_SWCResUpPress_enum] -> MSA Speed Setting ON/2("VTQD_SWCResUpPress_enum  ")
  [VTQD_SWCSetDownPress_enum] -> MSA Speed Setting ON/3("VTQD_SWCSetDownPress_enum  ")
  Rem/1 -> Data Type Conversion/1
  Data Type Conversion/1 -> [VTQD_SetSpdDeltaLongFit_kph]  "VTQD_SetSpdDeltaLongFit_kph"
  [VTQD_SetSpd_kph] -> Delay/1
  Delay/1 -> Rem/1
  Constant12/1 -> Rem/2
  [VTQD_SetSpdDeltaLongFit_kph] -> CC Speed Setting ON/5(VTQD_SetSpdDeltaLongFit_kph)
  [VVMC_MeterIndSpeed_raw32] -> CC Speed Setting ON/4(VVMC_MeterIndSpeed_raw32)
  [VVMC_MeterIndSpeed_raw32] -> MSA Speed Setting ON/4(VVMC_MeterIndSpeed_raw32)
  [VTQD_SetSpdDeltaLongFit_kph] -> MSA Speed Setting ON/5(VTQD_SetSpdDeltaLongFit_kph)
  Constant13/1 -> Else Speed Setting On/1(In)
  Else Speed Setting On/1(Out) -> [VTQD_ElseSetSpd_kph]
  [VTQD_ElseSetSpd_kph] -> Switch4/3
  [VINP_ADASACCSta_enum] -> ACC Speed Setting ON/7(VINP_ADASACCSta_enum)
  [VTQD_SWCResUpSta_flg] -> ACC Speed Setting ON/1(VTQD_SWCResUpSta_flg)
  VVMC_ACCObjDist_m/1 -> ACC Speed Setting ON/5(VVMC_ACCObjDist_m)
  [VTQD_SWCSetDownSta_flg] -> ACC Speed Setting ON/2(VTQD_SWCSetDownSta_flg)
  [VVMC_MeterIndSpeed_raw32] -> ACC Speed Setting ON/6(VVMC_MeterIndSpeed_raw32)
  [task_time_s] -> ACC Speed Setting ON/3(task_time_s)
  ACC Speed Setting ON/1(VTQD_ACCSetSpd_kph) -> VTQD_SWCACCSetSpd_kph/1, [VTQD_ACCSetSpd_kph]  "VTQD_SWCACCSetSpd_kph"
  VVMC_LVDAACCStatusInformation_flg/1 -> ACC Speed Setting ON/4(VVMC_LVDAACCStatusInformation_flg)
  VVMC_MeterIndSpeed_raw32/1 -> [VVMC_MeterIndSpeed_raw32]
  VINP_Distanceunit_flg/1 -> [VINP_Distanceunit_flg]
  [VINP_Distanceunit_flg] -> ACC Speed Setting ON/8(VINP_Distanceunit_flg)
  [VINP_Distanceunit_flg] -> CC Speed Setting ON/6(VINP_Distanceunit_flg)
  [VINP_Distanceunit_flg] -> MSA Speed Setting ON/6(VINP_Distanceunit_flg)
  VINP_SmartEcoModeSW_flg/1 -> [VINP_SmartEcoModeSW_flg]
  [VINP_SmartEcoModeSW_flg] -> ISA Speed Setting ON/2(VINP_SmartEcoModeSW_flg)
  [VINP_SmartEcoModeSW_flg] -> MSA Speed Setting ON/7(VINP_SmartEcoModeSW_flg)
  [VINP_SmartEcoModeSW_flg] -> CC Speed Setting ON/7(VINP_SmartEcoModeSW_flg)
  [VINP_SmartEcoModeSW_flg] -> ACC Speed Setting ON/9(VINP_SmartEcoModeSW_flg)
  VVMC_SetACCDisableAPS_flg/1 -> ACC Speed Setting ON/10(VVMC_SetACCDisableAPS_flg)
  Constant16/1 -> Switch6/3
  Constant18/1 -> Switch7/3
  [VTQD_SWCSetDownSta_flg] -> OR/2
  [VTQD_SWCResUpSta_flg] -> OR/1
  [VVMC_MeterIndSpeed_raw32] -> Relational Operator1/1
  [VTQD_SetSpd_kph] -> Relational Operator/1
  [VINP_Distanceunit_flg] -> Switch7/2
  AND7/1 -> AND8/1
  [VINP_Distanceunit_flg] -> Switch6/2
  Constant17/1 -> Switch6/1
  Switch5/1 -> Relational Operator/2
  [VINP_Distanceunit_flg] -> Switch5/2
  [VTQD_SetSpd_kph] -> Relational Operator2/1
  Constant15/1 -> Switch5/1
  Constant14/1 -> Switch5/3
  Relational Operator1/1 -> AND6/1
  Constant19/1 -> Switch7/1
  Relational Operator2/1 -> AND6/3
  Switch7/1 -> Relational Operator2/2
  [VINP_SmartEcoModeSW_flg] -> AND8/2
  Switch6/1 -> Relational Operator1/2
  Relational Operator/1 -> AND/1
  AND/1 -> AND7/1
  AND6/1 -> AND7/2
  AND8/1 -> VTQD_SetSpdLimWarn_flg/1  "VTQD_SetSpdLimWarn_flg"
  OR/1 -> AND6/2
  [VTQD_SWCResUpSta_flg] -> AND/2
  ACC Speed Setting ON/2(VTQD_SWCAllowSetSpd_flg) -> VTQD_SWCAllowSetSpd_flg/1
  CC Speed Setting ON/2(VTQD_SWCCCSpdResetFinish_flg) -> VTQD_SWCCCSpdResetFinish_flg/1

== system tqd/TQD/TorqueDemand/Signal_convert/SWC_Subsystem/VTQD_IVIISAOffsetSpdCHOOSE_flg ==
  VTQD_IVIISAOffsetSpd_enum : Inport
  Constant : Constant  Value=ENUM_IVIISAOFFSETSPD_MIUNS10KPH
  Constant1 : Constant  Value=ENUM_IVIISAOFFSETSPD_MIUNS5KPH
  Constant2 : Constant  Value=ENUM_IVIISAOFFSETSPD_0KPH
  Constant3 : Constant  Value=ENUM_IVIISAOFFSETSPD_PLUS5KPH
  Constant4 : Constant  Value=ENUM_IVIISAOFFSETSPD_PLUS10KPH
  Constant5 : Constant  Value=ENUM_IVIISAOFFSETSPD_MIUNS5MPH
  Constant6 : Constant  Value=ENUM_IVIISAOFFSETSPD_0MPH
  Constant7 : Constant  Value=ENUM_IVIISAOFFSETSPD_PLUS5MPH
  Constant8 : Constant  Value=TRUE
  Constant9 : Constant  Value=FALSE
  Equal{,1..7} (8 alike) : RelationalOperator  Operator===  OutDataTypeStr=boolean  RndMeth=Simplest
  OR : Logic  Operator=OR  Inputs=8  AllPortsSameDT=off  OutDataTypeStr=boolean
  Switch : Switch  Criteria=u2 ~= 0
  VTQD_IVIISAOffsetSpdCHOOSE_flg : Outport
  wires:
  VTQD_IVIISAOffsetSpd_enum/1 -> [VTQD_IVIISAOffsetSpd_enum], Equal/1
  Constant/1 -> Equal/2
  Equal/1 -> OR/1
  Constant1/1 -> Equal1/2
  Equal1/1 -> OR/2
  Equal2/1 -> OR/3
  Constant2/1 -> Equal2/2
  Constant5/1 -> Equal5/2
  Equal5/1 -> OR/6
  Equal4/1 -> OR/5
  Constant4/1 -> Equal4/2
  Equal3/1 -> OR/4
  Constant3/1 -> Equal3/2
  Equal6/1 -> OR/7
  Constant6/1 -> Equal6/2
  Constant7/1 -> Equal7/2
  Equal7/1 -> OR/8
  OR/1 -> Switch/2
  Constant8/1 -> Switch/1
  Constant9/1 -> Switch/3
  Switch/1 -> VTQD_IVIISAOffsetSpdCHOOSE_flg/1  "VTQD_IVIISAOffsetSpdCHOOSE_flg"
  [VTQD_IVIISAOffsetSpd_enum] -> Equal1/1
  [VTQD_IVIISAOffsetSpd_enum] -> Equal2/1
  [VTQD_IVIISAOffsetSpd_enum] -> Equal4/1
  [VTQD_IVIISAOffsetSpd_enum] -> Equal6/1
  [VTQD_IVIISAOffsetSpd_enum] -> Equal5/1
  [VTQD_IVIISAOffsetSpd_enum] -> Equal7/1
  [VTQD_IVIISAOffsetSpd_enum] -> Equal3/1

== system tqd/TQD/TorqueDemand/Signal_convert/SWC_Subsystem/Vehicle to Meter Speed ==
  InputSpeed : Inport
  Add : Sum
  Constant1 : Constant  Value=KTQD_Veh2MetSpdAdd_kph
  Constant11 : Constant  Value=KTQD_Veh2MetSpdGain_c
  Product : Product
  OutputSpeed : Outport
  wires:
  Constant1/1 -> Add/2
  Add/1 -> OutputSpeed/1
  Constant11/1 -> Product/2
  Product/1 -> Add/1
  InputSpeed/1 -> Product/1

== system tqd/TQD/TorqueDemand/Signal_convert/VehWeightEst/Calaulation ==
  task_time_s : Inport
  VTQD_VehWeightEstEn_flg : Inport  Port=2
  VTQD_VehWeightEstDis_flg : Inport  Port=3
  VTQD_VehWeightEstEnd_flg : Inport  Port=4
  VVMC_LongAcc_Gps : Inport  Port=5
  VINP_FrEDURealTMTq_Nm : Inport  Port=6
  VINP_RrEDURealTMTq_Nm : Inport  Port=7
  VINP_VehSpeed_kph : Inport  Port=8
  Front Wheel Torque : Subsystem
  Long Acc : Subsystem
  Rear Wheel Torque : Subsystem
  Vehicle Weight : Subsystem
  VTQD_EstLongAccCheckPass_flg : Outport
  VTQD_EstFrRealTqCheckPass_flg : Outport  Port=2
  VTQD_EstRrRealTqCheckPass_flg : Outport  Port=3
  VTQD_EstVehWeight_kg : Outport  Port=4
  wires:
  task_time_s/1 -> [task_time_s]
  VTQD_VehWeightEstEn_flg/1 -> [VTQD_VehWeightEstEn_flg]
  [VVMC_LongAcc_Gps] -> Long Acc/1(VVMC_LongAcc_Gps)
  [VTQD_VehWeightEstEn_flg] -> Long Acc/2(VTQD_VehWeightEstEn_flg)
  [VTQD_VehWeightEstDis_flg] -> Long Acc/3(VTQD_VehWeightEstDis_flg)
  [VTQD_VehWeightEstEnd_flg] -> Long Acc/4(VTQD_VehWeightEstEnd_flg)
  [task_time_s] -> Long Acc/5(task_time_s)
  [VINP_FrEDURealTMTq_Nm] -> Front Wheel Torque/1(VINP_FrEDURealTMTq_Nm)
  [VTQD_VehWeightEstEn_flg] -> Front Wheel Torque/2(VTQD_VehWeightEstEn_flg)
  [VTQD_VehWeightEstDis_flg] -> Front Wheel Torque/3(VTQD_VehWeightEstDis_flg)
  [VTQD_VehWeightEstEnd_flg] -> Front Wheel Torque/4(VTQD_VehWeightEstEnd_flg)
  [task_time_s] -> Front Wheel Torque/5(task_time_s)
  [VINP_RrEDURealTMTq_Nm] -> Rear Wheel Torque/1(VINP_RrEDURealTMTq_Nm)
  [VTQD_VehWeightEstEn_flg] -> Rear Wheel Torque/2(VTQD_VehWeightEstEn_flg)
  [VTQD_VehWeightEstDis_flg] -> Rear Wheel Torque/3(VTQD_VehWeightEstDis_flg)
  [VTQD_VehWeightEstEnd_flg] -> Rear Wheel Torque/4(VTQD_VehWeightEstEnd_flg)
  [task_time_s] -> Rear Wheel Torque/5(task_time_s)
  VTQD_VehWeightEstDis_flg/1 -> [VTQD_VehWeightEstDis_flg]
  VTQD_VehWeightEstEnd_flg/1 -> [VTQD_VehWeightEstEnd_flg]
  VVMC_LongAcc_Gps/1 -> [VVMC_LongAcc_Gps]
  VINP_FrEDURealTMTq_Nm/1 -> [VINP_FrEDURealTMTq_Nm]
  VINP_RrEDURealTMTq_Nm/1 -> [VINP_RrEDURealTMTq_Nm]
  Long Acc/1(VTQD_EstLongAccAvg_Gps) -> [VTQD_EstLongAccAvg_Gps]
  Long Acc/2(VTQD_EstLongAccCheckPass_flg) -> [VTQD_EstLongAccCheckPass_flg]
  Front Wheel Torque/1(VTQD_EstFrRealTqAvg_Nm) -> [VTQD_EstFrRealTqAvg_Nm]
  Front Wheel Torque/2(VTQD_EstFrRealTqCheckPass_flg) -> [VTQD_EstFrRealTqCheckPass_flg]
  Rear Wheel Torque/1(VTQD_EstRrRealTqAvg_Nm) -> [VTQD_EstRrRealTqAvg_Nm]
  Rear Wheel Torque/2(VTQD_EstRrRealTqCheckPass_flg) -> [VTQD_EstRrRealTqCheckPass_flg]
  [VTQD_EstLongAccCheckPass_flg] -> VTQD_EstLongAccCheckPass_flg/1
  [VTQD_EstRrRealTqCheckPass_flg] -> VTQD_EstRrRealTqCheckPass_flg/1
  [VTQD_EstFrRealTqCheckPass_flg] -> VTQD_EstFrRealTqCheckPass_flg/1
  [VTQD_EstFrRealTqAvg_Nm] -> Vehicle Weight/1(VTQD_EstFrRealTqAvg_Nm)
  [VTQD_EstRrRealTqAvg_Nm] -> Vehicle Weight/2(VTQD_EstRrRealTqAvg_Nm)
  [VTQD_EstLongAccAvg_Gps] -> Vehicle Weight/3(VTQD_EstLongAccAvg_Gps)
  [VINP_VehSpeed_kph] -> Vehicle Weight/4(VINP_VehSpeed_kph)
  VINP_VehSpeed_kph/1 -> [VINP_VehSpeed_kph]
  Vehicle Weight/1(VTQD_EstVehWeight_kg) -> [VTQD_EstVehWeight_kg]
  [VTQD_EstVehWeight_kg] -> VTQD_EstVehWeight_kg/1

== system tqd/TQD/TorqueDemand/Signal_convert/VehWeightEst/Condition ==
  VTQD_AfterAvailableTqDemRr_Nm : Inport
  VTQR_NoABSREDUWhlTqReq_Nm : Inport  Port=2
  VTQR_NoABSFEDUWhlTqReq_Nm : Inport  Port=3
  VTQD_AfterAvailableTqDemFr_Nm : Inport  Port=4
  VTQD_GearActualPosn_enum : Inport  Port=5
  VINP_VehSpeed_kph : Inport  Port=6
  VTQD_RollRegenDisableReq_flg : Inport  Port=7
  VINP_RegenMode_enum : Inport  Port=8
  VTQD_LowIdleAccPedal_flg : Inport  Port=9
  VTQD_BrkSwSta_flg : Inport  Port=10
  VINP_RrRBCActive_flg : Inport  Port=11
  VINP_FrRBCActive_flg : Inport  Port=12
  VINP_GRADE_Deg : Inport  Port=13
  task_time_s : Inport  Port=14
  VTQD_VehWeightEstEnd_flg : Inport  Port=15
  AND1 : Logic  Inputs=13  AllPortsSameDT=off  OutDataTypeStr=boolean
  Abs : Abs
  Abs1 : Abs
  Abs2 : Abs
  Add : Sum  Inputs=+-
  Add1 : Sum  Inputs=+-
  Constant1 : Constant  Value=KTQD_VehWeightEstSpdEnLow_kph
  Constant10 : Constant  Value=eps
  Constant11 : Constant  Value=KTQD_VehWeightEstSpdEnUp_kph
  Constant2 : Constant  Value=ENUM_REGENLEVEL_LV1
  Constant3 : Constant  Value=KTQD_RrTqDeviation_Nm
  Constant4 : Constant  Value=KTQD_FrTqDeviation_Nm
  Constant5 : Constant  Value=KTQD_VehWeightEstGradeEn_Deg
  Constant6 : Constant  Value=KTQD_VehWeighEstTime_s
  Constant7 : Constant  Value=KTQD_EstDelayEnTime_s
  Constant8 : Constant  Value=KTQD_EstWeighResetTime_s
  Constant9 : Constant  Value=ENUM_GEARACTUALPOSN_D
  Delay{,1..5} (6 alike) : Delay  DelayLength=1
  DelayEnable : hcu_lib/Basic_Blocks/DelayEnable
  Detect Increase : simulink/Logic and Bit Operations/Detect Increase  vinit=0.0  OutDataTypeStr=boolean
  Equal : RelationalOperator  Operator=<  OutDataTypeStr=boolean  RndMeth=Simplest
  Equal1 : RelationalOperator  Operator===  OutDataTypeStr=boolean  RndMeth=Simplest
  Equal2 : RelationalOperator  Operator=~=  OutDataTypeStr=boolean  RndMeth=Simplest
  Less Than1 : RelationalOperator  Operator=<  OutDataTypeStr=boolean  RndMeth=Simplest
  Less Than2 : RelationalOperator  Operator=>  OutDataTypeStr=boolean  RndMeth=Simplest
  Less Than3 : RelationalOperator  Operator=<=  OutDataTypeStr=boolean  RndMeth=Simplest
  Less Than4 : RelationalOperator  Operator=<=  OutDataTypeStr=boolean  RndMeth=Simplest
  Less Than5 : RelationalOperator  Operator=<=  OutDataTypeStr=boolean  RndMeth=Simplest
  NOT{,1..5} (6 alike) : Logic  Operator=NOT  AllPortsSameDT=off  OutDataTypeStr=boolean
  Relational Operator : RelationalOperator  OutDataTypeStr=boolean  RndMeth=Simplest
  Relational Operator1 : RelationalOperator  OutDataTypeStr=boolean  RndMeth=Simplest
  SR_Latch : hcu_lib/Basic_Blocks/SR_Latch
  Timer : hcu_lib/Basic_Blocks/Timer
  Timer1 : hcu_lib/Basic_Blocks/Timer
  VTQD_VehWeightEstEn_flg : Outport
  VTQD_VehWeightEstDis_flg : Outport  Port=2
  wires:
  Constant9/1 -> Equal1/2
  Less Than1/1 -> AND1/2  "VTQD_VehWeightEstEnCon2_flg"
  Abs/1 -> [VTQD_RrTqErr_Nm]  "VTQD_RrTqErr_Nm"
  Equal1/1 -> AND1/1  "VTQD_VehWeightEstEnCon1_flg"
  Constant11/1 -> Less Than1/2
  [VTQR_NoABSFEDUWhlTqReq_Nm] -> Delay1/1
  Constant4/1 -> Less Than4/2
  Add1/1 -> Abs1/1
  [VTQD_RollRegenDisableReq_flg] -> NOT/1
  [VTQD_RrTqErr_Nm] -> Less Than3/1
  Add/1 -> Abs/1
  [VTQD_BrkSwSta_flg] -> NOT3/1
  [VTQD_FrTqErr_Nm] -> Less Than4/1
  Abs1/1 -> [VTQD_FrTqErr_Nm]  "VTQD_FrTqErr_Nm"
  [VTQD_GearActualPosn_enum] -> Equal1/1
  [VINP_VehSpeed_kph] -> Less Than1/1
  [VINP_RegenMode_enum] -> Equal2/1
  [VTQD_AfterAvailableTqDemFr_Nm] -> Delay4/1
  Constant1/1 -> Less Than2/2
  [VTQD_AfterAvailableTqDemRr_Nm] -> Delay2/1
  Less Than4/1 -> AND1/8  "VTQD_VehWeightEstEnCon7_flg"
  [VINP_RrRBCActive_flg] -> NOT4/1
  [VTQR_NoABSREDUWhlTqReq_Nm] -> Delay3/1
  NOT/1 -> AND1/4  "VTQD_VehWeightEstEnCon4_flg"
  [VINP_FrRBCActive_flg] -> NOT5/1
  Constant5/1 -> Less Than5/2
  Equal2/1 -> AND1/5  "VTQD_VehWeightEstEnCon5_flg"
  [VTQD_LowIdleAccPedal_flg] -> AND1/6
  Constant2/1 -> Equal2/2
  Less Than3/1 -> AND1/7  "VTQD_VehWeightEstEnCon6_flg"
  Less Than2/1 -> AND1/3  "VTQD_VehWeightEstEnCon3_flg"
  [VINP_VehSpeed_kph] -> Less Than2/1
  Less Than5/1 -> AND1/12  "VTQD_VehWeightEstEnCon11_flg"
  [VINP_GRADE_Deg] -> Abs2/1
  Abs2/1 -> Less Than5/1
  Constant3/1 -> Less Than3/2
  VTQD_AfterAvailableTqDemRr_Nm/1 -> [VTQD_AfterAvailableTqDemRr_Nm]
  VTQR_NoABSREDUWhlTqReq_Nm/1 -> [VTQR_NoABSREDUWhlTqReq_Nm]
  VTQD_AfterAvailableTqDemFr_Nm/1 -> [VTQD_AfterAvailableTqDemFr_Nm]
  VTQR_NoABSFEDUWhlTqReq_Nm/1 -> [VTQR_NoABSFEDUWhlTqReq_Nm]
  VTQD_GearActualPosn_enum/1 -> [VTQD_GearActualPosn_enum]
  VINP_VehSpeed_kph/1 -> [VINP_VehSpeed_kph]
  VTQD_RollRegenDisableReq_flg/1 -> [VTQD_RollRegenDisableReq_flg]
  VINP_RegenMode_enum/1 -> [VINP_RegenMode_enum]
  VTQD_LowIdleAccPedal_flg/1 -> [VTQD_LowIdleAccPedal_flg]
  VTQD_BrkSwSta_flg/1 -> [VTQD_BrkSwSta_flg]
  VINP_RrRBCActive_flg/1 -> [VINP_RrRBCActive_flg]
  VINP_FrRBCActive_flg/1 -> [VINP_FrRBCActive_flg]
  VINP_GRADE_Deg/1 -> [VINP_GRADE_Deg]
  [VTQD_VehWeightEstEn_flg] -> VTQD_VehWeightEstEn_flg/1
  Relational Operator/1 -> [VTQD_VehWeightEstDis_flg]  "VTQD_VehWeightEstDis_flg"
  Timer/1 -> Relational Operator/1
  NOT1/1 -> Timer/2
  [VTQD_VehWeightEstEn_flg] -> NOT1/1, Timer/1
  Constant6/1 -> Relational Operator/2, Timer/4
  [VTQD_VehWeightEstDis_flg] -> VTQD_VehWeightEstDis_flg/1
  task_time_s/1 -> [task_time_s]
  AND1/1 -> DelayEnable/1
  DelayEnable/1 -> [VTQD_VehWeightEstEn_flg]  "VTQD_VehWeightEstEn_flg"
  [task_time_s] -> DelayEnable/3
  Constant7/1 -> DelayEnable/2
  [VTQD_VehWeightEstEnd_flg] -> Detect Increase/1
  Detect Increase/1 -> SR_Latch/1
  SR_Latch/1 -> NOT2/1, Timer1/1
  NOT2/1 -> Timer1/2
  Constant8/1 -> Relational Operator1/2, Timer1/4
  Timer1/1 -> [VTQD_EstVehWeightResetTime_s], Relational Operator1/1  "VTQD_EstVehWeightResetTime_s"
  Relational Operator1/1 -> [VTQD_EstVehWeitResetFinish_flg]  "VTQD_EstVehWeitResetFinish_flg"
  [VTQD_EstVehWeitResetFinish_flg] -> Delay/1
  Delay/1 -> SR_Latch/2
  [VTQD_EstVehWeightResetTime_s] -> Delay5/1
  Constant10/1 -> Equal/2
  Equal/1 -> AND1/13  "VTQD_VehWeightEstEnCon12_flg"
  VTQD_VehWeightEstEnd_flg/1 -> [VTQD_VehWeightEstEnd_flg]
  Delay1/1 -> Add1/1
  Delay2/1 -> Add/1
  Delay3/1 -> Add/2
  Delay4/1 -> Add1/2
  Delay5/1 -> Equal/1
  NOT3/1 -> AND1/9  "VTQD_VehWeightEstEnCon8_flg"
  NOT4/1 -> AND1/10  "VTQD_VehWeightEstEnCon9_flg"
  NOT5/1 -> AND1/11  "VTQD_VehWeightEstEnCon10_flg"
  [task_time_s] -> Timer/3
  [task_time_s] -> Timer1/3
